simulink model "Target_Control_System"  (R2021b)
settings: Solver=FixedStepDiscrete  StartTime=0.0  StopTime=5  RelTol=1e-3
PreLoadFcn:
  | RTWConfigurationCB('preloadfcn', bdroot);
PostLoadFcn:
  | load('configuration/data_struct.mat');
  | load('configuration/fluxMaps_propMotor.mat');
  | load('configuration/parameterInit_PROP.mat');
  | load('configuration/parameterInit_PUMP.mat');
  | load('configuration/parameterInit_PITCH.mat');
  | load('configuration/parameterInit_TILT.mat');
  | %load('configuration/base_workspace_signal_definition.mat');
  | %load('resolvedatastores_to_baseworkspace_for_faster_simulation.mat');
model workspace (MAT data in the model file):
  SIMULATION_OPTIONS : Simulink.Parameter (value not decoded)
  TARGET_CODE_GEN : Simulink.Parameter (value not decoded)
  TCS_SAMPLE_FREQ_HZ : Simulink.Parameter (value not decoded)
symbols that are objects in the model workspace (value not decoded): TARGET_CODE_GEN, TCS_SAMPLE_FREQ_HZ
undefined symbols (not defined in the file): A_DQ_REF_LPF_INIT__PITCH, A_DQ_REF_LPF_INIT__PROP, A_DQ_REF_LPF_INIT__PUMP, A_DQ_REF_LPF_INIT__TILT, A_OBSERVER_CONFIDENCE_INIT__PITCH, A_OBSERVER_CONFIDENCE_INIT__PROP, A_OBSERVER_CONFIDENCE_INIT__PUMP, A_OBSERVER_CONFIDENCE_INIT__TILT, ACTUATOR_MAX_ANGLE_TRIP__PITCH, ACTUATOR_MIN_ANGLE_TRIP__PITCH, ACTUATOR_POS_SENSOR_INV_DIRECTION__PITCH, ACTUATOR_POS_SENSOR_INV_DIRECTION__TILT, ACTUATOR_POS_SENSOR_OFFSET__PITCH, ACTUATOR_POS_SENSOR_OFFSET__TILT, ADC_scaler1_baseaddr_TILT, ADC_SCALER_FLOAT_TO_FIXPOINT_EXPANSION, ANGLE_ELEC_FROM_SENSOR_OFFSET_INIT__PITCH, ANGLE_ELEC_FROM_SENSOR_OFFSET_INIT__PROP, ANGLE_ELEC_FROM_SENSOR_OFFSET_INIT__PUMP, ANGLE_ELEC_FROM_SENSOR_OFFSET_INIT__TILT, AUTO_CLEAR_FAULTS_ENABLED__PITCH, AUTO_CLEAR_FAULTS_ENABLED__PROP, AUTO_CLEAR_FAULTS_ENABLED__PUMP, AUTO_CLEAR_FAULTS_ENABLED__TILT, AUTO_CLEAR_FAULTS_WAIT_TICKS__PITCH, AUTO_CLEAR_FAULTS_WAIT_TICKS__PROP, AUTO_CLEAR_FAULTS_WAIT_TICKS__PUMP, AUTO_CLEAR_FAULTS_WAIT_TICKS__TILT, AUTO_I_ZERO_IDLE_TICKS__PITCH, AUTO_I_ZERO_IDLE_TICKS__PROP, AUTO_I_ZERO_IDLE_TICKS__PUMP, AUTO_I_ZERO_IDLE_TICKS__TILT, AUTO_I_ZERO_OFFSET_IDC_THRESHOLD__PITCH, AUTO_I_ZERO_OFFSET_IDC_THRESHOLD__PROP, AUTO_I_ZERO_OFFSET_IDC_THRESHOLD__PUMP, AUTO_I_ZERO_OFFSET_IDC_THRESHOLD__TILT, AUTO_I_ZERO_OFFSET_IPH_THRESHOLD__PITCH, AUTO_I_ZERO_OFFSET_IPH_THRESHOLD__PROP, AUTO_I_ZERO_OFFSET_IPH_THRESHOLD__PUMP, AUTO_I_ZERO_OFFSET_IPH_THRESHOLD__TILT, AUTO_SENSORLESS_SWITCHOVER_DISABLE_OMEGA, AUTO_SENSORLESS_SWITCHOVER_ENABLE_OMEGA, AUTO_SENSORLESS_SWITCHOVER_MIN_CONFIDENCE, AUXILIARY_PROTECTION_UNIT_BASEADDR__TILT, blanking_max_error_omega_INIT_PITCH, blanking_max_error_omega_INIT_TILT, blanking_max_error_position_INIT_PITCH, blanking_max_error_position_INIT_TILT, BRUTE_START_I_Q_REF_RAMP_SPEED__PITCH, BRUTE_START_I_Q_REF_RAMP_SPEED__PROP, BRUTE_START_I_Q_REF_RAMP_SPEED__PUMP, BRUTE_START_I_Q_REF_RAMP_SPEED__TILT, CONTROL_LOOP_DT_INIT__PITCH, CONTROL_LOOP_DT_INIT__PROP, CONTROL_LOOP_DT_INIT__PUMP, CONTROL_LOOP_DT_INIT__TILT, CORRECTION_FILTER_SCALE__PITCH, CORRECTION_FILTER_SCALE__PROP, CORRECTION_FILTER_SCALE__PUMP, CORRECTION_FILTER_SCALE__TILT ... (+458)
libraries: simulink x178, Reusables_Lib x24
(part 25 of 47)

== system Target_Control_System/Target_Control_System/InterruptFunction/pitchMotor_isrTask/abcToAlphaBeta/Calc Angle From Speed/Integrator with Angle Wrapper ==
  Omega : Inport
  Add : Sum  Commented=on  Inputs=+-
  Add1 : Sum  Commented=on
  Add5 : Sum
  Add6 : Sum  Inputs=+-
  Add7 : Sum
  Constant1 : Constant  Commented=on  Value=2*pi  OutDataTypeStr=single  SampleTime=-1
  Constant11 : Constant  Commented=on  Value=-pi  OutDataTypeStr=single  SampleTime=-1
  Constant12 : Constant  Value=pi  OutDataTypeStr=single  SampleTime=-1
  Constant13 : Constant  Value=-pi  OutDataTypeStr=single  SampleTime=-1
  Constant14 : Constant  Value=2*pi  OutDataTypeStr=single  SampleTime=-1
  Constant15 : Constant  Value=2*pi  OutDataTypeStr=single  SampleTime=-1
  Constant2 : Constant  Commented=on  Value=2*pi  OutDataTypeStr=single  SampleTime=-1
  Constant6 : Constant  Commented=on  Value=pi  OutDataTypeStr=single  SampleTime=-1
  Data Store Read1 : DataStoreRead  DataStoreName=oPitch  DataStoreElements=oPitch.oIsr_.oParam_.fControlLoopDt_  IndexOptions=Index vector (dialog)  Indices=1  OutputSizes=1
  Data Store Read29 : DataStoreRead  Commented=on  DataStoreName=oProp  DataStoreElements=oProp.oIsr_.oParam_.fControlLoopDt_  IndexOptions=Index vector (dialog)  Indices=1  OutputSizes=1
  Discrete-Time Integrator4 : DiscreteIntegrator  Commented=on  IntegratorMethod=Accumulation: Forward Euler  ExternalReset=rising  InitialConditionSource=external  SampleTime=-1  ShowStatePort=on  ICPrevOutput=DiscIntNeverNeededParam  ICPrevScaledInput=DiscIntNeverNeededParam
  Equal3 : RelationalOperator  Commented=on  Operator=>  OutDataTypeStr=boolean  RndMeth=Simplest
  Equal4 : RelationalOperator  Commented=on  Operator=<  OutDataTypeStr=boolean  RndMeth=Simplest
  Equal5 : RelationalOperator  Operator=>  OutDataTypeStr=boolean  RndMeth=Simplest
  Equal6 : RelationalOperator  Operator=<  OutDataTypeStr=boolean  RndMeth=Simplest
  Logical Operator : Logic  Commented=on  Operator=OR  AllPortsSameDT=off  OutDataTypeStr=boolean
  Logical Operator2 : Logic  Operator=OR  AllPortsSameDT=off  OutDataTypeStr=boolean
  Product1 : Product
  Product16 : Product  Commented=on
  Switch1 : Switch  Commented=on  Criteria=u2 > Threshold  Threshold=0.5
  Switch2 : Switch  Commented=on  Criteria=u2 > Threshold  Threshold=0.5
  Switch5 : Switch  Criteria=u2 > Threshold
  Switch6 : Switch  Criteria=u2 > Threshold  Threshold=0.5
  Switch7 : Switch  Criteria=u2 > Threshold  Threshold=0.5
  Unit Delay1 : UnitDelay  SampleTime=-1  HasFrameUpgradeWarning=on
  Angle : Outport
  wires:
  Switch6/1 -> Switch7/3
  Omega/1 -> Product1/1
  Switch7/1 -> Switch5/1
  Add5/1 -> Switch5/3, Equal5/1, Equal6/1, Add7/1, Add6/1, Switch6/3
  Constant12/1 -> Equal5/2
  Logical Operator2/1 -> Switch5/2
  Unit Delay1/1 -> Add5/1
  Constant15/1 -> Add7/2
  Equal6/1 -> Switch7/2, Logical Operator2/2
  Add6/1 -> Switch6/1
  Product1/1 -> Add5/2
  Data Store Read1/1 -> Product1/2
  Add7/1 -> Switch7/1
  Equal5/1 -> Switch6/2, Logical Operator2/1
  Switch5/1 -> Unit Delay1/1, Angle/1
  Constant13/1 -> Equal6/2
  Constant14/1 -> Add6/2
  Data Store Read29/1 -> Product16/2
  Add/1 -> Switch2/1
  Switch2/1 -> Switch1/3
  Add1/1 -> Switch1/1
  Constant2/1 -> Add1/2
  Constant1/1 -> Add/2
  Equal3/1 -> Switch2/2, Logical Operator/1
  Switch1/1 -> Discrete-Time Integrator4/3
  Constant11/1 -> Equal4/2
  Logical Operator/1 -> Discrete-Time Integrator4/2
  Constant6/1 -> Equal3/2
  Product16/1 -> Discrete-Time Integrator4/1
  Equal4/1 -> Switch1/2, Logical Operator/2
  Discrete-Time Integrator4/State -> Add1/1, Equal4/1, Add/1, Switch2/3, Equal3/1

== system Target_Control_System/Target_Control_System/InterruptFunction/pitchMotor_isrTask/abcToAlphaBeta/Calc Angle From Speed/Integrator with Angle Wrapper_OLD ==
  Omega : Inport
  Add : Sum  Inputs=+-
  Add1 : Sum
  Constant1 : Constant  Value=2*pi  OutDataTypeStr=single  SampleTime=-1
  Constant11 : Constant  Value=-pi  OutDataTypeStr=single  SampleTime=-1
  Constant2 : Constant  Value=2*pi  OutDataTypeStr=single  SampleTime=-1
  Constant6 : Constant  Value=pi  OutDataTypeStr=single  SampleTime=-1
  Discrete-Time Integrator4 : DiscreteIntegrator  ExternalReset=rising  InitialConditionSource=external  SampleTime=-1  ShowStatePort=on  ICPrevOutput=DiscIntNeverNeededParam  ICPrevScaledInput=DiscIntNeverNeededParam
  Equal3 : RelationalOperator  Operator=>  OutDataTypeStr=boolean  RndMeth=Simplest
  Equal4 : RelationalOperator  Operator=<  OutDataTypeStr=boolean  RndMeth=Simplest
  Logical Operator : Logic  Operator=OR  AllPortsSameDT=off  OutDataTypeStr=boolean
  Switch1 : Switch  Criteria=u2 > Threshold  Threshold=0.5
  Switch2 : Switch  Criteria=u2 > Threshold  Threshold=0.5
  Angle : Outport
  wires:
  Add/1 -> Switch2/1
  Switch2/1 -> Switch1/3
  Add1/1 -> Switch1/1
  Constant2/1 -> Add1/2
  Constant1/1 -> Add/2
  Equal3/1 -> Switch2/2, Logical Operator/1
  Switch1/1 -> Discrete-Time Integrator4/3
  Constant11/1 -> Equal4/2
  Discrete-Time Integrator4/1 -> Angle/1
  Logical Operator/1 -> Discrete-Time Integrator4/2
  Constant6/1 -> Equal3/2
  Omega/1 -> Discrete-Time Integrator4/1
  Equal4/1 -> Switch1/2, Logical Operator/2
  Discrete-Time Integrator4/State -> Add1/1, Equal4/1, Add/1, Switch2/3, Equal3/1

== system Target_Control_System/Target_Control_System/InterruptFunction/pitchMotor_isrTask/abcToAlphaBeta/ModelSource/DoNotIncludeCustomCode ==

== system Target_Control_System/Target_Control_System/InterruptFunction/pitchMotor_isrTask/abcToAlphaBeta/ModelSource/IncludeCustomCode ==
  System Update : Subsystem  mask(System Update){ShowInLibBrowser=0}
      mask prompts: ShowInLibBrowser "Simulink:masks:CustCodeMaskParam1_MP"
      settings: CopyFcn=cccopyfcn(gcb)  OpenFcn=ccopenfcn('System Update Function')
      mask Help: eval('feval(''rtwprivate'',''rtwhelpview'',''rtw_sys_update_block'')');
      mask DialogControl ShowInLibBrowser Prompt: Mask Parameter 1:
      mask Display: disp('System\nUpdate');

== system Target_Control_System/Target_Control_System/InterruptFunction/pitchMotor_isrTask/currentController/Current Controller/Flux Feed-forward ==
  fFluxMainMagnitudeLpf : Inport
  fFluxFeedforwardGainRampOut : Inport  Port=2
  fOneOverUdc : Inport  Port=3
  fUqRefPiContrib : Inport  Port=4
  mdl_tilt_fOmegaE : Inport  Port=5
  Divide : Product  Inputs=****
  Saturation : Saturate  UpperLimit=1.1  LowerLimit=-1.1
  Sum : Sum  Inputs=|++
  fUqRef : Outport
  wires:
  mdl_tilt_fOmegaE/1 -> Divide/1
  Sum/1 -> fUqRef/1
  fOneOverUdc/1 -> Divide/4
  fFluxFeedforwardGainRampOut/1 -> Divide/3
  fFluxMainMagnitudeLpf/1 -> Divide/2
  fUqRefPiContrib/1 -> Sum/2
  Saturation/1 -> Sum/1
  Divide/1 -> Saturation/1

== system Target_Control_System/Target_Control_System/InterruptFunction/pitchMotor_isrTask/currentController/Current Controller/Limit Voltage Vector ==
  fUdRef : Inport
  fMaximumVoltageVectorLengthSquared : Inport  Port=2
  fUqRef : Inport  Port=3
  Add : Sum
  Add1 : Sum  Inputs=-+
  Compute Alpha-Beta Refs : Subsystem  Commented=on
  Constant1 : Constant  Value=0  OutDataTypeStr=single  SampleTime=-1
  Divide1 : Product  Inputs=**
  Divide2 : Product  Inputs=**
  Divide3 : Product  Inputs=**
  GreaterThan : RelationalOperator  Operator=>  OutDataTypeStr=boolean  RndMeth=Simplest
  Max : MinMax  Function=max  Inputs=2
  Sign : Signum
  Sqrt : Sqrt  SaturateOnIntegerOverflow=on
  Switch : Switch  Criteria=u2 > Threshold
  fUqRef_out : Outport
  fUdRef_out : Outport  Port=2
  wires:
  Sqrt/1 -> Divide3/1
  Switch/1 -> fUqRef_out/1  "fUqRef"
  fUdRef/1 -> Divide2/2, Divide2/1, fUdRef_out/1  "UdRef"
  Add1/1 -> Max/2
  Add/1 -> GreaterThan/1  "fVectorLengthSquared"
  Sign/1 -> Divide3/2
  Divide3/1 -> Switch/1
  Divide2/1 -> Add/1, Add1/1  "UdRef*UdRef"
  Max/1 -> Sqrt/1
  fUqRef/1 -> Divide1/2, Divide1/1, Sign/1, Switch/3
  GreaterThan/1 -> Switch/2
  Divide1/1 -> Add/2
  fMaximumVoltageVectorLengthSquared/1 -> GreaterThan/2, Add1/2
  Constant1/1 -> Max/1

== system Target_Control_System/Target_Control_System/InterruptFunction/pitchMotor_isrTask/currentController/Current Controller/PI Id Current Controller ==
  fTarget : Inport
  fActual : Inport  Port=2
  fKp : Inport  Port=3
  fKi : Inport  Port=4
  fScale : Inport  Port=5
  fLoopDt : Inport  Port=6
  fIntMax : Inport  Port=7
  fOutMax : Inport  Port=8
  fIntMin : Inport  Port=9
  fOutMin : Inport  Port=10
  fState : Inport  Port=11
  Add : Sum  Inputs=|++
  Mux : Mux  Inputs=3
  Mux1 : Mux  Inputs=3
  PI Id Controller Pitch : Scope  Commented=on  NumInputPorts=6
  Product : Product
  Saturation Dynamic : simulink/Discontinuities/Saturation Dynamic  OutMin=[]  OutMax=[]  OutDataTypeStr=Inherit: Same as second input  OutDataType=fixdt(1, 16)  OutScaling=2^-10  DoSatur=off
  Saturation Dynamic1 : simulink/Discontinuities/Saturation Dynamic  OutMin=[]  OutMax=[]  OutDataTypeStr=Inherit: Same as second input  OutDataType=fixdt(1, 16)  OutScaling=2^-10  DoSatur=off
  Sum1 : Sum  Inputs=++|
  Sum22 : Sum  Inputs=-+|
  Unit Delay2 : UnitDelay  SampleTime=-1  HasFrameUpgradeWarning=on
  fError * fKi_ * fScale : Fcn  Expr=u(1)*u(2)*u(3)
  fError * fKp_ * fScale1 : Fcn  Expr=u(1)*u(2)*u(3)
  fOutput : Outport
  *fpState : Outport  Port=2
  wires:
  Sum22/1 -> Mux1/1, Mux/3, PI Id Controller Pitch/3  "fError"
  fError * fKi_ * fScale/1 -> Product/1
  fTarget/1 -> PI Id Controller Pitch/1, Sum22/2
  fActual/1 -> PI Id Controller Pitch/2, Sum22/1
  Saturation Dynamic/1 -> Unit Delay2/1  "*fpState"
  fError * fKp_ * fScale1/1 -> PI Id Controller Pitch/4, Sum1/1
  Sum1/1 -> Saturation Dynamic1/2  "fError"
  Saturation Dynamic1/1 -> PI Id Controller Pitch/6, fOutput/1
  Mux/1 -> fError * fKi_ * fScale/1
  fKp/1 -> Mux1/2
  fScale/1 -> Mux1/3, Mux/1
  fKi/1 -> Mux/2
  Mux1/1 -> fError * fKp_ * fScale1/1
  Product/1 -> Add/1
  fState/1 -> Add/2
  Add/1 -> Saturation Dynamic/2
  fIntMax/1 -> Saturation Dynamic/1
  fIntMin/1 -> Saturation Dynamic/3
  fOutMin/1 -> Saturation Dynamic1/3
  fOutMax/1 -> Saturation Dynamic1/1
  fLoopDt/1 -> Product/2
  Unit Delay2/1 -> Sum1/2, *fpState/1, PI Id Controller Pitch/5

== system Target_Control_System/Target_Control_System/InterruptFunction/pitchMotor_isrTask/currentController/Current Controller/PI Iq Current Controller ==
  fTarget : Inport
  fActual : Inport  Port=2
  fKp : Inport  Port=3
  fKi : Inport  Port=4
  fScale : Inport  Port=5
  fLoopDt : Inport  Port=6
  fIntMax : Inport  Port=7
  fOutMax : Inport  Port=8
  fIntMin : Inport  Port=9
  fOutMin : Inport  Port=10
  fState : Inport  Port=11
  Add : Sum  Inputs=|++
  Mux : Mux  Inputs=3
  Mux1 : Mux  Inputs=3
  PI Iq Controller Pitch : Scope  Commented=on  NumInputPorts=6
  Product : Product
  Saturation Dynamic : simulink/Discontinuities/Saturation Dynamic  OutMin=[]  OutMax=[]  OutDataTypeStr=Inherit: Same as second input  OutDataType=fixdt(1, 16)  OutScaling=2^-10  DoSatur=off
  Saturation Dynamic1 : simulink/Discontinuities/Saturation Dynamic  OutMin=[]  OutMax=[]  OutDataTypeStr=Inherit: Same as second input  OutDataType=fixdt(1, 16)  OutScaling=2^-10  DoSatur=off
  Sum1 : Sum  Inputs=++|
  Sum22 : Sum  Inputs=-+|
  Unit Delay2 : UnitDelay  SampleTime=-1  HasFrameUpgradeWarning=on
  fError * fKi_ * fScale : Fcn  Expr=u(1)*u(2)*u(3)
  fError * fKp_ * fScale1 : Fcn  Expr=u(1)*u(2)*u(3)
  fOutput : Outport
  *fpState : Outport  Port=2
  wires:
  Sum22/1 -> Mux1/1, Mux/3, PI Iq Controller Pitch/3  "fError"
  fError * fKi_ * fScale/1 -> Product/1
  fTarget/1 -> PI Iq Controller Pitch/1, Sum22/2  "fTarget"
  fActual/1 -> PI Iq Controller Pitch/2, Sum22/1  "fActual"
  Saturation Dynamic/1 -> Unit Delay2/1  "*fpState"
  fError * fKp_ * fScale1/1 -> PI Iq Controller Pitch/4, Sum1/1
  Sum1/1 -> Saturation Dynamic1/2  "fError"
  Saturation Dynamic1/1 -> PI Iq Controller Pitch/6, fOutput/1  "fOutput"
  Mux/1 -> fError * fKi_ * fScale/1
  fKp/1 -> Mux1/2
  fScale/1 -> Mux1/3, Mux/1
  fKi/1 -> Mux/2
  Mux1/1 -> fError * fKp_ * fScale1/1
  Product/1 -> Add/1
  fState/1 -> Add/2
  Add/1 -> Saturation Dynamic/2
  fIntMax/1 -> Saturation Dynamic/1
  fIntMin/1 -> Saturation Dynamic/3
  fOutMin/1 -> Saturation Dynamic1/3
  fOutMax/1 -> Saturation Dynamic1/1
  fLoopDt/1 -> Product/2
  Unit Delay2/1 -> Sum1/2, *fpState/1, PI Iq Controller Pitch/5  "fpState"

== system Target_Control_System/Target_Control_System/InterruptFunction/pitchMotor_isrTask/fluxAngleCalculations/Advance Forced Angle/Integrator with Angle Wrapper ==
  Omega : Inport
  Add : Sum  Commented=on  Inputs=+-
  Add1 : Sum  Commented=on
  Add5 : Sum
  Add6 : Sum  Inputs=+-
  Add7 : Sum
  Constant1 : Constant  Commented=on  Value=2*pi  OutDataTypeStr=single  SampleTime=-1
  Constant11 : Constant  Commented=on  Value=-pi  OutDataTypeStr=single  SampleTime=-1
  Constant12 : Constant  Value=pi  OutDataTypeStr=single  SampleTime=-1
  Constant13 : Constant  Value=-pi  OutDataTypeStr=single  SampleTime=-1
  Constant14 : Constant  Value=2*pi  OutDataTypeStr=single  SampleTime=-1
  Constant15 : Constant  Value=2*pi  OutDataTypeStr=single  SampleTime=-1
  Constant2 : Constant  Commented=on  Value=2*pi  OutDataTypeStr=single  SampleTime=-1
  Constant6 : Constant  Commented=on  Value=pi  OutDataTypeStr=single  SampleTime=-1
  Data Store Read1 : DataStoreRead  DataStoreName=oPitch  DataStoreElements=oPitch.oIsr_.oParam_.fControlLoopDt_  IndexOptions=Index vector (dialog)  Indices=1  OutputSizes=1
  Data Store Read29 : DataStoreRead  Commented=on  DataStoreName=oProp  DataStoreElements=oProp.oIsr_.oParam_.fControlLoopDt_  IndexOptions=Index vector (dialog)  Indices=1  OutputSizes=1
  Discrete-Time Integrator4 : DiscreteIntegrator  Commented=on  IntegratorMethod=Accumulation: Forward Euler  ExternalReset=rising  InitialConditionSource=external  SampleTime=-1  ShowStatePort=on  ICPrevOutput=DiscIntNeverNeededParam  ICPrevScaledInput=DiscIntNeverNeededParam
  Equal3 : RelationalOperator  Commented=on  Operator=>  OutDataTypeStr=boolean  RndMeth=Simplest
  Equal4 : RelationalOperator  Commented=on  Operator=<  OutDataTypeStr=boolean  RndMeth=Simplest
  Equal5 : RelationalOperator  Operator=>  OutDataTypeStr=boolean  RndMeth=Simplest
  Equal6 : RelationalOperator  Operator=<  OutDataTypeStr=boolean  RndMeth=Simplest
  Logical Operator : Logic  Commented=on  Operator=OR  AllPortsSameDT=off  OutDataTypeStr=boolean
  Logical Operator2 : Logic  Operator=OR  AllPortsSameDT=off  OutDataTypeStr=boolean
  Product1 : Product
  Product16 : Product  Commented=on
  Switch1 : Switch  Commented=on  Criteria=u2 > Threshold  Threshold=0.5
  Switch2 : Switch  Commented=on  Criteria=u2 > Threshold  Threshold=0.5
  Switch5 : Switch  Criteria=u2 > Threshold
  Switch6 : Switch  Criteria=u2 > Threshold  Threshold=0.5
  Switch7 : Switch  Criteria=u2 > Threshold  Threshold=0.5
  Unit Delay1 : UnitDelay  SampleTime=-1  HasFrameUpgradeWarning=on
  Angle : Outport
  wires:
  Switch6/1 -> Switch7/3
  Omega/1 -> Product1/1
  Switch7/1 -> Switch5/1
  Add5/1 -> Switch5/3, Equal5/1, Equal6/1, Add7/1, Add6/1, Switch6/3
  Constant12/1 -> Equal5/2
  Logical Operator2/1 -> Switch5/2
  Unit Delay1/1 -> Add5/1
  Constant15/1 -> Add7/2
  Equal6/1 -> Switch7/2, Logical Operator2/2
  Add6/1 -> Switch6/1
  Product1/1 -> Add5/2
  Data Store Read1/1 -> Product1/2
  Add7/1 -> Switch7/1
  Equal5/1 -> Switch6/2, Logical Operator2/1
  Switch5/1 -> Unit Delay1/1, Angle/1
  Constant13/1 -> Equal6/2
  Constant14/1 -> Add6/2
  Data Store Read29/1 -> Product16/2
  Add/1 -> Switch2/1
  Switch2/1 -> Switch1/3
  Add1/1 -> Switch1/1
  Constant2/1 -> Add1/2
  Constant1/1 -> Add/2
  Equal3/1 -> Switch2/2, Logical Operator/1
  Switch1/1 -> Discrete-Time Integrator4/3
  Constant11/1 -> Equal4/2
  Logical Operator/1 -> Discrete-Time Integrator4/2
  Constant6/1 -> Equal3/2
  Product16/1 -> Discrete-Time Integrator4/1
  Equal4/1 -> Switch1/2, Logical Operator/2
  Discrete-Time Integrator4/State -> Add1/1, Equal4/1, Add/1, Switch2/3, Equal3/1

== system Target_Control_System/Target_Control_System/InterruptFunction/pitchMotor_isrTask/fluxAngleCalculations/Advance Forced Angle/Integrator with Angle Wrapper_OLD ==
  Omega : Inport
  Add : Sum  Inputs=+-
  Add1 : Sum
  Constant1 : Constant  Value=2*pi  OutDataTypeStr=single  SampleTime=-1
  Constant11 : Constant  Value=-pi  OutDataTypeStr=single  SampleTime=-1
  Constant2 : Constant  Value=2*pi  OutDataTypeStr=single  SampleTime=-1
  Constant6 : Constant  Value=pi  OutDataTypeStr=single  SampleTime=-1
  Discrete-Time Integrator4 : DiscreteIntegrator  ExternalReset=rising  InitialConditionSource=external  SampleTime=-1  ShowStatePort=on  ICPrevOutput=DiscIntNeverNeededParam  ICPrevScaledInput=DiscIntNeverNeededParam
  Equal3 : RelationalOperator  Operator=>  OutDataTypeStr=boolean  RndMeth=Simplest
  Equal4 : RelationalOperator  Operator=<  OutDataTypeStr=boolean  RndMeth=Simplest
  Logical Operator : Logic  Operator=OR  AllPortsSameDT=off  OutDataTypeStr=boolean
  Switch1 : Switch  Criteria=u2 > Threshold  Threshold=0.5
  Switch2 : Switch  Criteria=u2 > Threshold  Threshold=0.5
  Angle : Outport
  wires:
  Add/1 -> Switch2/1
  Switch2/1 -> Switch1/3
  Add1/1 -> Switch1/1
  Constant2/1 -> Add1/2
  Constant1/1 -> Add/2
  Equal3/1 -> Switch2/2, Logical Operator/1
  Switch1/1 -> Discrete-Time Integrator4/3
  Constant11/1 -> Equal4/2
  Discrete-Time Integrator4/1 -> Angle/1
  Logical Operator/1 -> Discrete-Time Integrator4/2
  Constant6/1 -> Equal3/2
  Omega/1 -> Discrete-Time Integrator4/1
  Equal4/1 -> Switch1/2, Logical Operator/2
  Discrete-Time Integrator4/State -> Add1/1, Equal4/1, Add/1, Switch2/3, Equal3/1

== system Target_Control_System/Target_Control_System/InterruptFunction/pitchMotor_isrTask/fluxAngleCalculations/Back Rotation/Angle Clip ==
  Angle_In : Inport
  Add1 : Sum  Inputs=-+
  Add12 : Sum  Inputs=-+
  Add2 : Sum
  Add3 : Sum
  Equal1 : RelationalOperator  Operator=>  OutDataTypeStr=boolean  RndMeth=Simplest
  Equal2 : RelationalOperator  Operator=<  OutDataTypeStr=boolean  RndMeth=Simplest
  Equal3 : RelationalOperator  Operator=<  OutDataTypeStr=boolean  RndMeth=Simplest
  Equal5 : RelationalOperator  Operator=>  OutDataTypeStr=boolean  RndMeth=Simplest
  Pi : Constant  Value=pi  OutDataTypeStr=single  SampleTime=-1
  Pi1 : Constant  Value=2*pi  OutDataTypeStr=single  SampleTime=-1
  Pi2 : Constant  Value=-pi  OutDataTypeStr=single  SampleTime=-1
  Pi3 : Constant  Value=2*pi  OutDataTypeStr=single  SampleTime=-1
  Pi4 : Constant  Value=-pi  OutDataTypeStr=single  SampleTime=-1
  Pi8 : Constant  Value=pi  OutDataTypeStr=single  SampleTime=-1
  Switch{1..3,5} (4 alike) : Switch  Criteria=u2 > Threshold  Threshold=0.5
  Angle_Out : Outport
  wires:
  Switch3/1 -> Switch2/1
  Equal2/1 -> Switch3/2
  Switch5/1 -> Switch2/3, Add3/2, Equal3/1
  Add2/1 -> Switch3/1
  Pi3/1 -> Add3/1, Add2/1
  Add3/1 -> Switch3/3, Equal2/1, Add2/2
  Pi4/1 -> Equal2/2
  Switch2/1 -> Angle_Out/1
  Equal3/1 -> Switch2/2
  Pi2/1 -> Equal3/2
  Switch1/1 -> Switch5/1
  Add1/1 -> Switch1/1
  Equal5/1 -> Switch1/2
  Pi8/1 -> Equal5/2
  Add12/1 -> Equal5/1, Add1/2, Switch1/3
  Pi/1 -> Equal1/2
  Equal1/1 -> Switch5/2
  Angle_In/1 -> Add12/2, Equal1/1, Switch5/3
  Pi1/1 -> Add12/1, Add1/1

== system Target_Control_System/Target_Control_System/InterruptFunction/pitchMotor_isrTask/fluxAngleCalculations/ModelSource/DoNotIncludeCustomCode ==

== system Target_Control_System/Target_Control_System/InterruptFunction/pitchMotor_isrTask/fluxAngleCalculations/ModelSource/IncludeCustomCode ==
  System Update : Subsystem  mask(System Update){ShowInLibBrowser=0}
      mask prompts: ShowInLibBrowser "Simulink:masks:CustCodeMaskParam1_MP"
      settings: CopyFcn=cccopyfcn(gcb)  OpenFcn=ccopenfcn('System Update Function')
      mask Help: eval('feval(''rtwprivate'',''rtwhelpview'',''rtw_sys_update_block'')');
      mask DialogControl ShowInLibBrowser Prompt: Mask Parameter 1:
      mask Display: disp('System\nUpdate');

== system Target_Control_System/Target_Control_System/InterruptFunction/pitchMotor_isrTask/fluxAngleCalculations/Not forced Angle/Angle Clip ==
  Angle_In : Inport
  Add1 : Sum  Inputs=-+
  Add12 : Sum  Inputs=-+
  Add2 : Sum
  Add3 : Sum
  Equal1 : RelationalOperator  Operator=>  OutDataTypeStr=boolean  RndMeth=Simplest
  Equal2 : RelationalOperator  Operator=<  OutDataTypeStr=boolean  RndMeth=Simplest
  Equal3 : RelationalOperator  Operator=<  OutDataTypeStr=boolean  RndMeth=Simplest
  Equal5 : RelationalOperator  Operator=>  OutDataTypeStr=boolean  RndMeth=Simplest
  Pi : Constant  Value=pi  OutDataTypeStr=single  SampleTime=-1
  Pi1 : Constant  Value=2*pi  OutDataTypeStr=single  SampleTime=-1
  Pi2 : Constant  Value=-pi  OutDataTypeStr=single  SampleTime=-1
  Pi3 : Constant  Value=2*pi  OutDataTypeStr=single  SampleTime=-1
  Pi4 : Constant  Value=-pi  OutDataTypeStr=single  SampleTime=-1
  Pi8 : Constant  Value=pi  OutDataTypeStr=single  SampleTime=-1
  Switch{1..3,5} (4 alike) : Switch  Criteria=u2 > Threshold  Threshold=0.5
  Angle_Out : Outport
  wires:
  Switch3/1 -> Switch2/1
  Equal2/1 -> Switch3/2
  Switch5/1 -> Switch2/3, Add3/2, Equal3/1
  Add2/1 -> Switch3/1
  Pi3/1 -> Add3/1, Add2/1
  Add3/1 -> Switch3/3, Equal2/1, Add2/2
  Pi4/1 -> Equal2/2
  Switch2/1 -> Angle_Out/1
  Equal3/1 -> Switch2/2
  Pi2/1 -> Equal3/2
  Switch1/1 -> Switch5/1
  Add1/1 -> Switch1/1
  Equal5/1 -> Switch1/2
  Pi8/1 -> Equal5/2
  Add12/1 -> Equal5/1, Add1/2, Switch1/3
  Pi/1 -> Equal1/2
  Equal1/1 -> Switch5/2
  Angle_In/1 -> Add12/2, Equal1/1, Switch5/3
  Pi1/1 -> Add12/1, Add1/1

== system Target_Control_System/Target_Control_System/InterruptFunction/pitchMotor_isrTask/fluxObserver/Fast PLL/piControllerStep_fOmegaE_pitch ==
  fScale : Inport
  fActual : Inport  Port=2
  fTarget : Inport  Port=3
  fKp : Inport  Port=4
  fKi : Inport  Port=5
  fLoopDt : Inport  Port=6
  fIntMax : Inport  Port=7
  fOutMax : Inport  Port=8
  fIntMin : Inport  Port=9
  fOutMin : Inport  Port=10
  fState : Inport  Port=11
  Add : Sum  Inputs=|++
  Mux : Mux  Inputs=3
  Mux1 : Mux  Inputs=3
  Product : Product
  Saturation Dynamic : simulink/Discontinuities/Saturation Dynamic  OutMin=[]  OutMax=[]  OutDataTypeStr=Inherit: Same as second input  OutDataType=fixdt(1, 16)  OutScaling=2^-10  DoSatur=off
  Saturation Dynamic1 : simulink/Discontinuities/Saturation Dynamic  OutMin=[]  OutMax=[]  OutDataTypeStr=Inherit: Same as second input  OutDataType=fixdt(1, 16)  OutScaling=2^-10  DoSatur=off
  Scope3 : Scope  NumInputPorts=6
  Sum1 : Sum  Inputs=++|
  Sum22 : Sum  Inputs=-+|
  Unit Delay2 : UnitDelay  SampleTime=-1  HasFrameUpgradeWarning=on
  fError * fKi_ * fScale : Fcn  Expr=u(1)*u(2)*u(3)
  fError * fKp_ * fScale1 : Fcn  Expr=u(1)*u(2)*u(3)
  fOutput : Outport
  *fpState : Outport  Port=2
  wires:
  fLoopDt/1 -> Product/2
  fOutMax/1 -> Saturation Dynamic1/1
  fOutMin/1 -> Saturation Dynamic1/3
  fIntMin/1 -> Saturation Dynamic/3
  fIntMax/1 -> Saturation Dynamic/1
  Unit Delay2/1 -> Scope3/5, *fpState/1, Sum1/2
  Add/1 -> Saturation Dynamic/2
  fState/1 -> Add/2
  Product/1 -> Add/1
  Mux1/1 -> fError * fKp_ * fScale1/1
  fKi/1 -> Mux/2
  fScale/1 -> Mux/1, Mux1/3
  fKp/1 -> Mux1/2
  Mux/1 -> fError * fKi_ * fScale/1
  Saturation Dynamic1/1 -> fOutput/1, Scope3/6
  Sum1/1 -> Saturation Dynamic1/2  "fError"
  fError * fKp_ * fScale1/1 -> Sum1/1, Scope3/4
  Saturation Dynamic/1 -> Unit Delay2/1  "*fpState"
  fActual/1 -> Sum22/1, Scope3/2
  fTarget/1 -> Sum22/2, Scope3/1
  fError * fKi_ * fScale/1 -> Product/1
  Sum22/1 -> Scope3/3, Mux/3, Mux1/1  "fError"

== system Target_Control_System/Target_Control_System/InterruptFunction/pitchMotor_isrTask/pwmGeneration/Subsystem/ABC to DQ ==
  iInverseDirection : Inport
  UdRef : Inport  Port=2
  UqRef : Inport  Port=3
  fFluxMasterAngleBkwd_sin : Inport  Port=4
  fFluxMasterAngleBkwd_cos : Inport  Port=5
  Mux : Mux  Inputs=2
  Mux5 : Mux
  Switch1 : Switch  Criteria=u2 > Threshold
  alpha/beta to abc : Gain  Gain="[1  0; -0.5 sqrt(3)/2; -0.5 -sqrt(3)/2]"  Multiplication=Matrix(K*u) (u vector)
  alpha/beta to abc_inverseDirection : Gain  Gain="[1  0; -0.5 -sqrt(3)/2; -0.5 sqrt(3)/2]"  Multiplication=Matrix(K*u) (u vector)
  fUAlphaRef_ = afOutArray[3]*fUdRef - afOutArray[2]*fUqRef : Fcn  Expr=u(4)*u(1)-u(3)*u(2)
  fUBetaRef_ = afOutArray[3]*fUqRef + afOutArray[2]*fUdRef : Fcn  Expr=u(4)*u(2)+u(3)*u(1)
  U_abc : Outport
  wires:
  iInverseDirection/1 -> Switch1/2
  fFluxMasterAngleBkwd_cos/1 -> Mux5/4
  fFluxMasterAngleBkwd_sin/1 -> Mux5/3
  UdRef/1 -> Mux5/1
  fUBetaRef_ = afOutArray[3]*fUqRef + afOutArray[2]*fUdRef/1 -> Mux/2  "fUBetaRef_"
  Mux5/1 -> fUAlphaRef_ = afOutArray[3]*fUdRef - afOutArray[2]*fUqRef/1, fUBetaRef_ = afOutArray[3]*fUqRef + afOutArray[2]*fUdRef/1
  alpha/beta to abc/1 -> Switch1/3
  alpha/beta to abc_inverseDirection/1 -> Switch1/1
  Switch1/1 -> U_abc/1
  Mux/1 -> alpha/beta to abc_inverseDirection/1, alpha/beta to abc/1
  UqRef/1 -> Mux5/2
  fUAlphaRef_ = afOutArray[3]*fUdRef - afOutArray[2]*fUqRef/1 -> Mux/1  "fUAlphaRef_"

== system Target_Control_System/Target_Control_System/InterruptFunction/pitchMotor_isrTask/pwmGeneration/Subsystem/Calculate Duty Cycles ==
  fUaRef : Inport
  fUbRef : Inport  Port=2
  fUcRef : Inport  Port=3
  fMaximumDuty : Inport  Port=4
  fHalfPositiveDuty : Inport  Port=5
  fPwmPeriodTicksFloat : Inport  Port=6
  Constant1 : Constant  Value=0.5  OutDataTypeStr=single  SampleTime=-1
  Constant11 : Constant  Value=-1  SampleTime=-1
  Constant4 : Constant  Value=0.5  OutDataTypeStr=single  SampleTime=-1
  Constant6 : Constant  Value=0.5  OutDataTypeStr=single  SampleTime=-1
  Data Type Conversion : DataTypeConversion  OutDataTypeStr=uint32
  Data Type Conversion1 : DataTypeConversion  OutDataTypeStr=uint32
  Data Type Conversion2 : DataTypeConversion  OutDataTypeStr=uint32
  Product{1,6..10} (6 alike) : Product
  Saturation Dynamic : simulink/Discontinuities/Saturation Dynamic  OutMin=[]  OutMax=[]  OutDataTypeStr=Inherit: Same as second input  OutDataType=fixdt(1, 16)  OutScaling=2^-10  DoSatur=off
  Saturation Dynamic1 : simulink/Discontinuities/Saturation Dynamic  OutMin=[]  OutMax=[]  OutDataTypeStr=Inherit: Same as second input  OutDataType=fixdt(1, 16)  OutScaling=2^-10  DoSatur=off
  Saturation Dynamic2 : simulink/Discontinuities/Saturation Dynamic  OutMin=[]  OutMax=[]  OutDataTypeStr=Inherit: Same as second input  OutDataType=fixdt(1, 16)  OutScaling=2^-10  DoSatur=off
  Sum1 : Sum  Inputs=|++  OutDataTypeStr=single
  Sum4 : Sum  Inputs=|++  OutDataTypeStr=single
  Sum5 : Sum  Inputs=|++  OutDataTypeStr=single
  uiPwmDutyTicksA : Outport
  uiPwmDutyTicksB : Outport  Port=2
  uiPwmDutyTicksC : Outport  Port=3
  wires:
  Data Type Conversion2/1 -> uiPwmDutyTicksC/1
  Data Type Conversion1/1 -> uiPwmDutyTicksB/1
  Data Type Conversion/1 -> uiPwmDutyTicksA/1
  fMaximumDuty/1 -> Saturation Dynamic/1, Saturation Dynamic1/1, Saturation Dynamic2/1
  fHalfPositiveDuty/1 -> Product1/2, Product7/2, Product6/2
  fPwmPeriodTicksFloat/1 -> Product10/2, Product9/2, Product8/2
  Constant1/1 -> Sum1/2
  fUbRef/1 -> Saturation Dynamic1/2
  fUcRef/1 -> Saturation Dynamic2/2
  fUaRef/1 -> Saturation Dynamic/2
  Sum1/1 -> Product8/1
  Product9/1 -> Data Type Conversion1/1
  Constant6/1 -> Sum5/2
  Saturation Dynamic/1 -> Product1/1
  Product7/1 -> Sum5/1
  Sum5/1 -> Product10/1
  Constant4/1 -> Sum4/2
  Product1/1 -> Sum1/1
  Product6/1 -> Sum4/1
  Constant11/1 -> Saturation Dynamic/3, Saturation Dynamic1/3, Saturation Dynamic2/3
  Sum4/1 -> Product9/1
  Product8/1 -> Data Type Conversion/1
  Saturation Dynamic2/1 -> Product7/1
  Saturation Dynamic1/1 -> Product6/1
  Product10/1 -> Data Type Conversion2/1

== system Target_Control_System/Target_Control_System/InterruptFunction/pitchMotor_isrTask/pwmGeneration/Subsystem/Zero sequence injection ==
  U_abc : Inport
  Demux : Demux  Outputs=3
  Gain4 : Gain  Gain=0.5
  Max : MinMax  Function=max  Inputs=3
  Max1 : MinMax  Inputs=3
  Sum6 : Sum  OutDataTypeStr=single
  Sum7 : Sum  Inputs=|+-  OutDataTypeStr=single
  Sum8 : Sum  Inputs=|+-  OutDataTypeStr=single
  Sum9 : Sum  Inputs=|+-  OutDataTypeStr=single
  fUaRef : Outport
  fUbRef : Outport  Port=2
  fUcRef : Outport  Port=3
  wires:
  U_abc/1 -> Demux/1
  Demux/3 -> Max1/3, Max/3, Sum9/1  "Uc"
  Max/1 -> Sum6/1
  Sum9/1 -> fUcRef/1  "fUcRef"
  Sum7/1 -> fUaRef/1  "fUaRef"
  Gain4/1 -> Sum7/2, Sum8/2, Sum9/2  "fUOffCenter"
  Demux/2 -> Max1/1, Max/2, Sum8/1  "Ub"
  Sum8/1 -> fUbRef/1  "fUbRef"
  Max1/1 -> Sum6/2
  Sum6/1 -> Gain4/1  "Umax+Umin"
  Demux/1 -> Sum7/1, Max/1, Max1/2  "Ua"

== system Target_Control_System/Target_Control_System/InterruptFunction/pitchMotor_setPwm/ModelSourceFPGAPitch/IncludeCustomCode/System Update ==

== system Target_Control_System/Target_Control_System/InterruptFunction/propMotor_IsrSchedule/Isr_Variant/CodeGen_IsrEnable/manageSmallInverterCounter ==
  Trigger : TriggerPort  VariantControl=(inherit)  PortDimensions=1
  Add : Sum
  Constant : Constant  Value=0
  Data Store Read : DataStoreRead  DataStoreName=mdl_suiIsrSmallInvCounter_  IndexOptions=Index vector (dialog)  Indices=1  OutputSizes=1
  Data Store Write : DataStoreWrite  DataStoreName=fpga_uiPWMInterruptCount_  IndexOptions=Index vector (dialog)  Indices=1  OutputSizes=1
  Data Store Write1 : DataStoreWrite  DataStoreName=mdl_suiIsrSmallInvCounter_  IndexOptions=Index vector (dialog)  Indices=1  OutputSizes=1
  Function-Call Generator : simulink/Ports & Subsystems/Function-Call Generator  sample_time=-1  numberOfIterations=1  DisallowWideOutput=off
  Switch : Switch  Criteria=u2 > Threshold  Threshold=3
  constant1 : Constant  OutDataTypeStr=uint32  SampleTime=-1
  constant2 : Constant  Value=0  OutDataTypeStr=uint32  SampleTime=-1
  IsrEnable : Outport
  wires:
  Constant/1 -> Data Store Write/1
  Function-Call Generator/1 -> IsrEnable/1
  constant1/1 -> Add/2
  Switch/1 -> Data Store Write1/1
  Data Store Read/1 -> Add/1
  Add/1 -> Switch/2, Switch/3
  constant2/1 -> Switch/1

== system Target_Control_System/Target_Control_System/InterruptFunction/propMotor_isrTask/abcToAlphaBeta/ModelSourceFOProp/DoNotIncludeCustomCode ==

== system Target_Control_System/Target_Control_System/InterruptFunction/propMotor_isrTask/abcToAlphaBeta/ModelSourceFOProp/IncludeCustomCode ==
  System Update : Subsystem  mask(System Update){ShowInLibBrowser=0}
      mask prompts: ShowInLibBrowser "Simulink:masks:CustCodeMaskParam1_MP"
      settings: CopyFcn=cccopyfcn(gcb)  OpenFcn=ccopenfcn('System Update Function')
      mask Help: eval('feval(''rtwprivate'',''rtwhelpview'',''rtw_sys_update_block'')');
      mask DialogControl ShowInLibBrowser Prompt: Mask Parameter 1:
      mask Display: disp('System\nUpdate');

== system Target_Control_System/Target_Control_System/InterruptFunction/propMotor_isrTask/currentController/Subsystem/Flux Feed-forward ==
  fUqRefPiContrib : Inport
  fFluxMainMagnitudeLpf : Inport  Port=2
  fFluxFeedforwardGainRampOut : Inport  Port=3
  fOneOverUdc : Inport  Port=4
  mdl_tilt_fOmegaE : Inport  Port=5
  Divide : Product  Inputs=****
  Saturation : Saturate  UpperLimit=1.1  LowerLimit=-1.1
  Sum : Sum  Inputs=|++
  fUqRef : Outport
  wires:
  mdl_tilt_fOmegaE/1 -> Divide/1
  Sum/1 -> fUqRef/1
  fOneOverUdc/1 -> Divide/4
  fFluxFeedforwardGainRampOut/1 -> Divide/3
  fFluxMainMagnitudeLpf/1 -> Divide/2
  fUqRefPiContrib/1 -> Sum/2
  Saturation/1 -> Sum/1
  Divide/1 -> Saturation/1

== system Target_Control_System/Target_Control_System/InterruptFunction/propMotor_isrTask/currentController/Subsystem/Limit Voltage Vector ==
  fUdRef : Inport
  fMaximumVoltageVectorLengthSquared : Inport  Port=2
  fUqRef : Inport  Port=3
  Add : Sum
  Divide1 : Product  Inputs=**
  Divide2 : Product  Inputs=**
  GreaterThan : RelationalOperator  Operator=>  OutDataTypeStr=boolean  RndMeth=Simplest
  Sign : Signum
  Subsystem : Subsystem
  Switch : Switch  Criteria=u2 > Threshold
  fUdRef_out : Outport
  fUqRef_out : Outport  Port=2
  wires:
  Sign/1 -> Subsystem/3(In3)
  GreaterThan/1 -> Subsystem/Enable, Switch/2
  Divide1/1 -> Add/1  "UqRef*UqRef"
  Subsystem/1(Out1) -> Switch/1
  Switch/1 -> fUqRef_out/1  "fUqRef"
  fUdRef/1 -> Divide2/1, Divide2/2, fUdRef_out/1  "UdRef"
  Add/1 -> GreaterThan/1  "fVectorLengthSquared"
  Divide2/1 -> Subsystem/2(UdRef*UdRef), Add/2  "UdRef*UdRef"
  fUqRef/1 -> Sign/1, Switch/3, Divide1/2, Divide1/1
  fMaximumVoltageVectorLengthSquared/1 -> GreaterThan/2, Subsystem/1(fMaximumVoltageVectorLengthSquared_)

== system Target_Control_System/Target_Control_System/InterruptFunction/propMotor_isrTask/currentController/Subsystem/PI Id Current Controller ==
  fActual : Inport
  fTarget : Inport  Port=2
  fKp : Inport  Port=3
  fKi : Inport  Port=4
  fScale : Inport  Port=5
  fLoopDt : Inport  Port=6
  fIntMax : Inport  Port=7
  fOutMax : Inport  Port=8
  fIntMin : Inport  Port=9
  fOutMin : Inport  Port=10
  fState : Inport  Port=11
  Add : Sum  Inputs=|++
  Mux : Mux  Inputs=3
  Mux1 : Mux  Inputs=3
  Product : Product
  Saturation Dynamic : simulink/Discontinuities/Saturation Dynamic  OutMin=[]  OutMax=[]  OutDataTypeStr=Inherit: Same as second input  OutDataType=fixdt(1, 16)  OutScaling=2^-10  DoSatur=on
  Saturation Dynamic1 : simulink/Discontinuities/Saturation Dynamic  OutMin=[]  OutMax=[]  OutDataTypeStr=Inherit: Same as second input  OutDataType=fixdt(1, 16)  OutScaling=2^-10  DoSatur=on
  Scope3 : Scope  NumInputPorts=6
  Sum1 : Sum  Inputs=++|
  Sum22 : Sum  Inputs=-+|
  fError * fKi_ * fScale : Fcn  Expr=u(1)*u(2)*u(3)
  fError * fKp_ * fScale1 : Fcn  Expr=u(1)*u(2)*u(3)
  fOutput : Outport
  *fpState : Outport  Port=2
  wires:
  fIntMin/1 -> Saturation Dynamic/3
  fLoopDt/1 -> Product/2
  fOutMax/1 -> Saturation Dynamic1/1
  fOutMin/1 -> Saturation Dynamic1/3
  fIntMax/1 -> Saturation Dynamic/1
  Add/1 -> Saturation Dynamic/2
  fState/1 -> Add/2
  Product/1 -> Add/1
  Mux1/1 -> fError * fKp_ * fScale1/1
  fKi/1 -> Mux/2
  fScale/1 -> Mux/1, Mux1/3
  fKp/1 -> Mux1/2
  Mux/1 -> fError * fKi_ * fScale/1
  Saturation Dynamic1/1 -> fOutput/1, Scope3/6
  Sum1/1 -> Saturation Dynamic1/2  "fError"
  fError * fKp_ * fScale1/1 -> Sum1/1, Scope3/4
  Saturation Dynamic/1 -> Scope3/5, *fpState/1, Sum1/2  "*fpState"
  fActual/1 -> Sum22/1, Scope3/2
  fTarget/1 -> Sum22/2, Scope3/1
  fError * fKi_ * fScale/1 -> Product/1
  Sum22/1 -> Scope3/3, Mux/3, Mux1/1  "fError"

== system Target_Control_System/Target_Control_System/InterruptFunction/propMotor_isrTask/currentController/Subsystem/PI Iq Current Controller ==
  fActual : Inport
  fTarget : Inport  Port=2
  fKp : Inport  Port=3
  fKi : Inport  Port=4
  fScale : Inport  Port=5
  fLoopDt : Inport  Port=6
  fIntMax : Inport  Port=7
  fOutMax : Inport  Port=8
  fIntMin : Inport  Port=9
  fOutMin : Inport  Port=10
  fState : Inport  Port=11
  Add : Sum  Inputs=|++
  Mux : Mux  Inputs=3
  Mux1 : Mux  Inputs=3
  Product : Product
  Saturation Dynamic : simulink/Discontinuities/Saturation Dynamic  OutMin=[]  OutMax=[]  OutDataTypeStr=Inherit: Same as second input  OutDataType=fixdt(1, 16)  OutScaling=2^-10  DoSatur=on
  Saturation Dynamic1 : simulink/Discontinuities/Saturation Dynamic  OutMin=[]  OutMax=[]  OutDataTypeStr=Inherit: Same as second input  OutDataType=fixdt(1, 16)  OutScaling=2^-10  DoSatur=on
  Scope3 : Scope  NumInputPorts=6
  Sum1 : Sum  Inputs=++|
  Sum22 : Sum  Inputs=-+|
  fError * fKi_ * fScale : Fcn  Expr=u(1)*u(2)*u(3)
  fError * fKp_ * fScale1 : Fcn  Expr=u(1)*u(2)*u(3)
  fOutput : Outport
  *fpState : Outport  Port=2
  wires:
  fIntMax/1 -> Saturation Dynamic/1
  fLoopDt/1 -> Product/2
  fOutMax/1 -> Saturation Dynamic1/1
  fOutMin/1 -> Saturation Dynamic1/3
  fIntMin/1 -> Saturation Dynamic/3
  Add/1 -> Saturation Dynamic/2
  fState/1 -> Add/2
  Product/1 -> Add/1
  Mux1/1 -> fError * fKp_ * fScale1/1
  fKi/1 -> Mux/2
  fScale/1 -> Mux/1, Mux1/3
  fKp/1 -> Mux1/2
  Mux/1 -> fError * fKi_ * fScale/1
  Saturation Dynamic1/1 -> fOutput/1, Scope3/6
  Sum1/1 -> Saturation Dynamic1/2  "fError"
  fError * fKp_ * fScale1/1 -> Sum1/1, Scope3/4
  Saturation Dynamic/1 -> Scope3/5, *fpState/1, Sum1/2  "*fpState"
  fActual/1 -> Sum22/1, Scope3/2
  fTarget/1 -> Sum22/2, Scope3/1
  fError * fKi_ * fScale/1 -> Product/1
  Sum22/1 -> Scope3/3, Mux/3, Mux1/1  "fError"

== system Target_Control_System/Target_Control_System/InterruptFunction/propMotor_isrTask/currentController/Subsystem/Subsystem ==
  Enable : EnablePort
  Add : Sum  Inputs=+-
  Constant : Constant  Value=0  OutDataTypeStr=single  SampleTime=-1
  Constant1 : Constant  Value=0  OutDataTypeStr=single  SampleTime=-1
  Data Store Read1 : DataStoreRead  DataStoreName=oProp  DataStoreElements=oProp.oIsr_.oParam_.fOverspeedProtectionDownstep_  IndexOptions=Index vector (dialog)  Indices=1  OutputSizes=1
  Data Store Read18 : DataStoreRead  DataStoreName=oProp  DataStoreElements=oProp.oIsr_.oState_.fOverspeedProtectionScaler_  IndexOptions=Index vector (dialog)  Indices=1  OutputSizes=1
  Data Store Write8 : DataStoreWrite  DataStoreName=oProp  DataStoreElements=oProp.oIsr_.oState_.fOverspeedProtectionScaler_  IndexOptions=Index vector (dialog)  Indices=1  OutputSizes=1
  Equal : RelationalOperator  Operator=<  OutDataTypeStr=boolean  RndMeth=Simplest
  Switch : Switch  Criteria=u2 > Threshold
  Output : Outport
  wires:
  Constant1/1 -> Switch/1
  Constant/1 -> Equal/2
  Equal/1 -> Switch/2
  Add/1 -> Switch/3, Equal/1
  Switch/1 -> Data Store Write8/1, Output/1
  Data Store Read18/1 -> Add/1
  Data Store Read1/1 -> Add/2

== system Target_Control_System/Target_Control_System/InterruptFunction/propMotor_isrTask/currentController/Subsystem/Subsystem1 ==
  note: fOverspeedProtectionScaler_
  Enable : EnablePort
  Add : Sum
  Constant : Constant  OutDataTypeStr=single  SampleTime=-1
  Constant1 : Constant  OutDataTypeStr=single  SampleTime=-1
  Data Store Read1 : DataStoreRead  DataStoreName=oProp  DataStoreElements=oProp.oIsr_.oParam_.fOverspeedProtectionUpstep_  IndexOptions=Index vector (dialog)  Indices=1  OutputSizes=1
  Data Store Read18 : DataStoreRead  DataStoreName=oProp  DataStoreElements=oProp.oIsr_.oState_.fOverspeedProtectionScaler_  IndexOptions=Index vector (dialog)  Indices=1  OutputSizes=1
  Data Store Write8 : DataStoreWrite  DataStoreName=oProp  DataStoreElements=oProp.oIsr_.oState_.fOverspeedProtectionScaler_  IndexOptions=Index vector (dialog)  Indices=1  OutputSizes=1
  Equal : RelationalOperator  Operator=>  OutDataTypeStr=boolean  RndMeth=Simplest
  Switch : Switch  Criteria=u2 > Threshold
  Output : Outport
  wires:
  Constant1/1 -> Switch/1
  Constant/1 -> Equal/2
  Equal/1 -> Switch/2
  Add/1 -> Switch/3, Equal/1
  Switch/1 -> Data Store Write8/1, Output/1
  Data Store Read18/1 -> Add/1
  Data Store Read1/1 -> Add/2

== system Target_Control_System/Target_Control_System/InterruptFunction/propMotor_isrTask/fluxAngleCalculation/ModelSource/DoNotIncludeCustomCode ==

== system Target_Control_System/Target_Control_System/InterruptFunction/propMotor_isrTask/fluxAngleCalculation/ModelSource/IncludeCustomCode ==
  System Update : Subsystem  mask(System Update){ShowInLibBrowser=0}
      mask prompts: ShowInLibBrowser "Simulink:masks:CustCodeMaskParam1_MP"
      settings: CopyFcn=cccopyfcn(gcb)  OpenFcn=ccopenfcn('System Update Function')
      mask Help: eval('feval(''rtwprivate'',''rtwhelpview'',''rtw_sys_update_block'')');
      mask DialogControl ShowInLibBrowser Prompt: Mask Parameter 1:
      mask Display: disp('System\nUpdate');

== system Target_Control_System/Target_Control_System/InterruptFunction/propMotor_isrTask/fluxAngleCalculation/Subsystem/Integrator with Angle Wrapper ==
  Omega : Inport
  Add : Sum  Commented=on  Inputs=+-
  Add1 : Sum  Commented=on
  Add5 : Sum
  Add6 : Sum  Inputs=+-
  Add7 : Sum
  Constant1 : Constant  Commented=on  Value=2*pi  OutDataTypeStr=single  SampleTime=-1
  Constant11 : Constant  Commented=on  Value=-pi  OutDataTypeStr=single  SampleTime=-1
  Constant12 : Constant  Value=pi  OutDataTypeStr=single  SampleTime=-1
  Constant13 : Constant  Value=-pi  OutDataTypeStr=single  SampleTime=-1
  Constant14 : Constant  Value=2*pi  OutDataTypeStr=single  SampleTime=-1
  Constant15 : Constant  Value=2*pi  OutDataTypeStr=single  SampleTime=-1
  Constant2 : Constant  Commented=on  Value=2*pi  OutDataTypeStr=single  SampleTime=-1
  Constant6 : Constant  Commented=on  Value=pi  OutDataTypeStr=single  SampleTime=-1
  Data Store Read1 : DataStoreRead  DataStoreName=oProp  DataStoreElements=oProp.oIsr_.oParam_.fControlLoopDt_  IndexOptions=Index vector (dialog)  Indices=1  OutputSizes=1
  Data Store Read29 : DataStoreRead  Commented=on  DataStoreName=oProp  DataStoreElements=oProp.oIsr_.oParam_.fControlLoopDt_  IndexOptions=Index vector (dialog)  Indices=1  OutputSizes=1
  Discrete-Time Integrator4 : DiscreteIntegrator  Commented=on  IntegratorMethod=Accumulation: Forward Euler  ExternalReset=rising  InitialConditionSource=external  SampleTime=-1  ShowStatePort=on  ICPrevOutput=DiscIntNeverNeededParam  ICPrevScaledInput=DiscIntNeverNeededParam
  Equal3 : RelationalOperator  Commented=on  Operator=>  OutDataTypeStr=boolean  RndMeth=Simplest
  Equal4 : RelationalOperator  Commented=on  Operator=<  OutDataTypeStr=boolean  RndMeth=Simplest
  Equal5 : RelationalOperator  Operator=>  OutDataTypeStr=boolean  RndMeth=Simplest
  Equal6 : RelationalOperator  Operator=<  OutDataTypeStr=boolean  RndMeth=Simplest
  Logical Operator : Logic  Commented=on  Operator=OR  AllPortsSameDT=off  OutDataTypeStr=boolean
  Logical Operator2 : Logic  Operator=OR  AllPortsSameDT=off  OutDataTypeStr=boolean
  Product1 : Product
  Product16 : Product  Commented=on
  Switch1 : Switch  Commented=on  Criteria=u2 > Threshold  Threshold=0.5
  Switch2 : Switch  Commented=on  Criteria=u2 > Threshold  Threshold=0.5
  Switch5 : Switch  Criteria=u2 > Threshold
  Switch6 : Switch  Criteria=u2 > Threshold  Threshold=0.5
  Switch7 : Switch  Criteria=u2 > Threshold  Threshold=0.5
  Unit Delay1 : UnitDelay  SampleTime=-1  HasFrameUpgradeWarning=on
  Angle : Outport
  wires:
  Switch6/1 -> Switch7/3
  Omega/1 -> Product1/1
  Switch7/1 -> Switch5/1
  Add5/1 -> Switch5/3, Equal5/1, Equal6/1, Add7/1, Add6/1, Switch6/3
  Constant12/1 -> Equal5/2
  Logical Operator2/1 -> Switch5/2
  Unit Delay1/1 -> Add5/1
  Constant15/1 -> Add7/2
  Equal6/1 -> Switch7/2, Logical Operator2/2
  Add6/1 -> Switch6/1
  Product1/1 -> Add5/2
  Data Store Read1/1 -> Product1/2
  Add7/1 -> Switch7/1
  Equal5/1 -> Switch6/2, Logical Operator2/1
  Switch5/1 -> Unit Delay1/1, Angle/1
  Constant13/1 -> Equal6/2
  Constant14/1 -> Add6/2
  Data Store Read29/1 -> Product16/2
  Add/1 -> Switch2/1
  Switch2/1 -> Switch1/3
  Add1/1 -> Switch1/1
  Constant2/1 -> Add1/2
  Constant1/1 -> Add/2
  Equal3/1 -> Switch2/2, Logical Operator/1
  Switch1/1 -> Discrete-Time Integrator4/3
  Constant11/1 -> Equal4/2
  Logical Operator/1 -> Discrete-Time Integrator4/2
  Constant6/1 -> Equal3/2
  Product16/1 -> Discrete-Time Integrator4/1
  Equal4/1 -> Switch1/2, Logical Operator/2
  Discrete-Time Integrator4/State -> Add1/1, Equal4/1, Add/1, Switch2/3, Equal3/1

== system Target_Control_System/Target_Control_System/InterruptFunction/propMotor_isrTask/fluxAngleCalculation/Subsystem/Integrator with Angle Wrapper_OLD ==
  Omega : Inport
  Add : Sum  Inputs=+-
  Add1 : Sum
  Constant1 : Constant  Value=2*pi  OutDataTypeStr=single  SampleTime=-1
  Constant11 : Constant  Value=-pi  OutDataTypeStr=single  SampleTime=-1
  Constant2 : Constant  Value=2*pi  OutDataTypeStr=single  SampleTime=-1
  Constant6 : Constant  Value=pi  OutDataTypeStr=single  SampleTime=-1
  Data Store Read29 : DataStoreRead  DataStoreName=oProp  DataStoreElements=oProp.oIsr_.oParam_.fControlLoopDt_  IndexOptions=Index vector (dialog)  Indices=1  OutputSizes=1
  Discrete-Time Integrator4 : DiscreteIntegrator  IntegratorMethod=Accumulation: Forward Euler  ExternalReset=rising  InitialConditionSource=external  SampleTime=-1  ShowStatePort=on  ICPrevOutput=DiscIntNeverNeededParam  ICPrevScaledInput=DiscIntNeverNeededParam
  Equal3 : RelationalOperator  Operator=>  OutDataTypeStr=boolean  RndMeth=Simplest
  Equal4 : RelationalOperator  Operator=<  OutDataTypeStr=boolean  RndMeth=Simplest
  Logical Operator : Logic  Operator=OR  AllPortsSameDT=off  OutDataTypeStr=boolean
  Product16 : Product
  Switch1 : Switch  Criteria=u2 > Threshold  Threshold=0.5
  Switch2 : Switch  Criteria=u2 > Threshold  Threshold=0.5
  Angle : Outport
  wires:
  Product16/1 -> Discrete-Time Integrator4/1
  Data Store Read29/1 -> Product16/2
  Omega/1 -> Product16/1
  Add/1 -> Switch2/1
  Switch2/1 -> Switch1/3
  Add1/1 -> Switch1/1
  Constant2/1 -> Add1/2
  Constant1/1 -> Add/2
  Equal3/1 -> Switch2/2, Logical Operator/1
  Switch1/1 -> Discrete-Time Integrator4/3
  Constant11/1 -> Equal4/2
  Discrete-Time Integrator4/1 -> Angle/1
  Logical Operator/1 -> Discrete-Time Integrator4/2
  Constant6/1 -> Equal3/2
  Equal4/1 -> Switch1/2, Logical Operator/2
  Discrete-Time Integrator4/State -> Add1/1, Equal4/1, Add/1, Switch2/3, Equal3/1

== system Target_Control_System/Target_Control_System/InterruptFunction/propMotor_isrTask/fluxAngleCalculation/Subsystem1/Angle Clip ==
  Angle_In : Inport
  Add1 : Sum  Inputs=-+
  Add12 : Sum  Inputs=-+
  Add2 : Sum
  Add3 : Sum
  Equal1 : RelationalOperator  Operator=>  OutDataTypeStr=boolean  RndMeth=Simplest
  Equal2 : RelationalOperator  Operator=<  OutDataTypeStr=boolean  RndMeth=Simplest
  Equal3 : RelationalOperator  Operator=<  OutDataTypeStr=boolean  RndMeth=Simplest
  Equal5 : RelationalOperator  Operator=>  OutDataTypeStr=boolean  RndMeth=Simplest
  Pi : Constant  Value=pi  OutDataTypeStr=single  SampleTime=-1
  Pi1 : Constant  Value=2*pi  OutDataTypeStr=single  SampleTime=-1
  Pi2 : Constant  Value=-pi  OutDataTypeStr=single  SampleTime=-1
  Pi3 : Constant  Value=2*pi  OutDataTypeStr=single  SampleTime=-1
  Pi4 : Constant  Value=-pi  OutDataTypeStr=single  SampleTime=-1
  Pi8 : Constant  Value=pi  OutDataTypeStr=single  SampleTime=-1
  Switch{1..3,5} (4 alike) : Switch  Criteria=u2 > Threshold  Threshold=0.5
  Angle_Out : Outport
  wires:
  Switch3/1 -> Switch2/1
  Equal2/1 -> Switch3/2
  Switch5/1 -> Switch2/3, Add3/2, Equal3/1
  Add2/1 -> Switch3/1
  Pi3/1 -> Add3/1, Add2/1
  Add3/1 -> Switch3/3, Equal2/1, Add2/2
  Pi4/1 -> Equal2/2
  Switch2/1 -> Angle_Out/1
  Equal3/1 -> Switch2/2
  Pi2/1 -> Equal3/2
  Switch1/1 -> Switch5/1
  Add1/1 -> Switch1/1
  Equal5/1 -> Switch1/2
  Pi8/1 -> Equal5/2
  Add12/1 -> Equal5/1, Add1/2, Switch1/3
  Pi/1 -> Equal1/2
  Equal1/1 -> Switch5/2
  Angle_In/1 -> Add12/2, Equal1/1, Switch5/3
  Pi1/1 -> Add12/1, Add1/1
